simulink model "RisingEdgeCounterWithReset"  (R2025a)
settings: Solver=VariableStepAuto  StartTime=0.0  StopTime=10.0  RelTol=1e-3
libraries: simulink x1
settings Model: Creator=mahij  LastModifiedBy=mahij

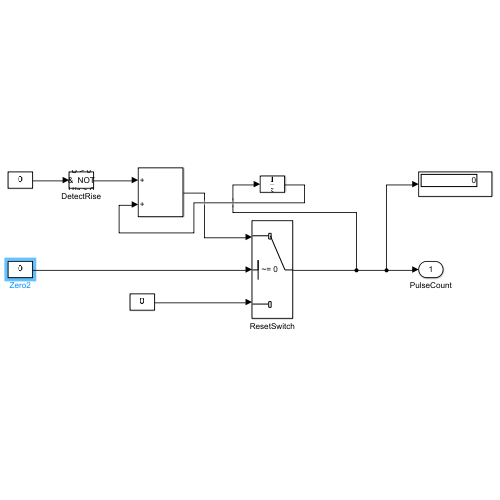
[thumbnail: Simulink's stored preview of the top-level diagram]
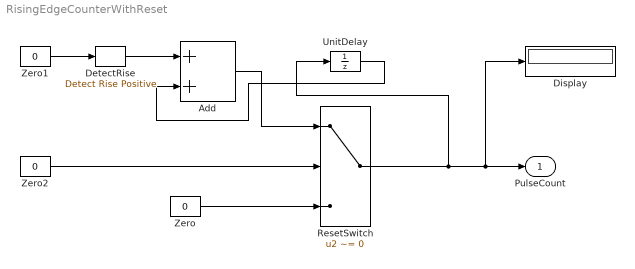
== system RisingEdgeCounterWithReset ==
  Add : Sum
  DetectRise : simulink/Logic and Bit Operations/Detect Rise Positive  vinit=0  OutDataTypeStr=boolean
  Display : Display
  ResetSwitch : Switch  Criteria=u2 ~= 0  Threshold=0.5  SaturateOnIntegerOverflow=off  InputSameDT=off
  UnitDelay : UnitDelay  SampleTime=-1  HasFrameUpgradeWarning=on
  Zero : Constant  Value=0
  Zero1 : Constant  Value=0
  Zero2 : Constant  Value=0
  PulseCount : Outport
  wires:
  Zero1/1 -> DetectRise/1
  DetectRise/1 -> Add/1
  UnitDelay/1 -> Add/2
  Add/1 -> ResetSwitch/1
  Zero2/1 -> ResetSwitch/2
  Zero/1 -> ResetSwitch/3
  ResetSwitch/1 -> UnitDelay/1, Display/1, PulseCount/1
